simulink model "problem3model"  (R2020a)
settings: Solver=ode45  StartTime=0.0  StopTime=25  MaxStep=0.1  RelTol=1e-3  AbsTol=1e-6
PostLoadFcn:
  | g = 32.18;
  | v0 = 88;
  | Rr = 15/12;  % Wheel radius
  | Kf = 1;
  | m = 50;
  | PBmax = 1500;
  | TB = 0.01;
  | I = 5;
undefined symbols (not defined in the file): mu, sigbuilder_block, slip
settings Model: Creator=Jake  LastModifiedBy=Jake

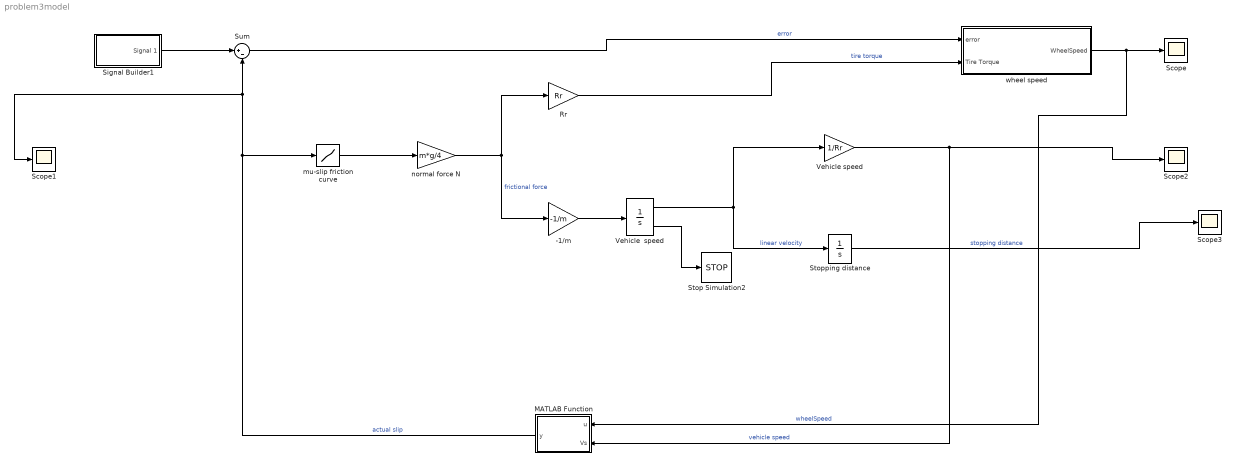
== system problem3model ==
  -1/m : Gain  Gain=-1/m  SaturateOnIntegerOverflow=on  OutDataTypeStr=Inherit: Same as input  ParamDataTypeStr=Inherit: Same as input
  MATLAB Function : MATLAB Function  TreatAsAtomicUnit=on
  Rr : Gain  Gain=Rr  SaturateOnIntegerOverflow=on  OutDataTypeStr=Inherit: Same as input  ParamDataTypeStr=Inherit: Same as input
  Scope{,1..3} (4 alike) : Scope
  Signal Builder1 : Subsystem  Tag=STV Subsys  LoadFcn=sigbuilder_block('load');  StartFcn=sigbuilder_block('start');  StopFcn=sigbuilder_block('stop');  ClipboardFcn=sigbuilder_block('clipboard');  mask(Sigbuilder block){tuvar=[0:10]}
      mask help: Simulink:masks:SigbuilderBlock_MD
      mask init:
      | if ~strcmp(get_param(bdroot(gcbh),'SimulationStatus'),'stopped') tuvar = sigbuilder_block('maskInit'); end
      settings: CopyFcn=sigbuilder_block('copy');  DeleteFcn=sigbuilder_block('delete');  ModelCloseFcn=sigbuilder_block('modelClose');  PreSaveFcn=sigbuilder_block('preSave');  PauseFcn=sigbuilder_block('pause');  ContinueFcn=sigbuilder_block('continue');  NameChangeFcn=sigbuilder_block('namechange');  OpenFcn=sigbuilder_block('open',[404 117.5 550.5 362.5 ]);  CloseFcn=sigbuilder_block('close');
      mask Display: plot(0, 0, 100, 100,[2, 2, 32, 32, 2], [68, 8, 8, 68, 68],[32, 2], [38, 38], [32, 19, 2],[53, 60, 44], [32, 17, 17, 2],[16, 16, 31, 31]);txt = getActiveGroup(gcbh);text(2, 100, txt,'verticalAlignment', 'top');
  Stop Simulation2 : Stop
  Stopping distance : Integrator  UpperSaturationLimit=1000  LowerSaturationLimit=0
  Sum : Sum  Inputs=|+-
  Vehicle  speed : Integrator  InitialCondition=v0  LimitOutput=on  UpperSaturationLimit=1000  LowerSaturationLimit=0  ShowSaturationPort=on
  Vehicle speed : Gain  Gain=1/Rr  SaturateOnIntegerOverflow=on  OutDataTypeStr=Inherit: Same as input  ParamDataTypeStr=Inherit: Same as input
  mu-slip friction curve : Lookup_n-D  NumberOfTableDimensions=1  BreakpointsForDimension1=slip  Table=mu  SaturateOnIntegerOverflow=on  InputSameDT=on
  normal force N : Gain  Gain=m*g/4
  wheel speed : Subsystem
  wires:
  Signal Builder1/1(Signal 1) -> Sum/1
  MATLAB Function/1(y) -> mu-slip friction curve/1, Scope1/1, Sum/2  "actual slip"
  normal force N/1 -> -1/m/1, Rr/1  "frictional force"
  -1/m/1 -> Vehicle  speed/1
  Vehicle  speed/2 -> Stop Simulation2/1
  Vehicle  speed/1 -> Stopping distance/1, Vehicle speed/1  "linear velocity"
  Stopping distance/1 -> Scope3/1  "stopping distance"
  mu-slip friction curve/1 -> normal force N/1
  Vehicle speed/1 -> MATLAB Function/2(Vs), Scope2/1  "vehicle speed"
  Sum/1 -> wheel speed/1(error)  "error"
  Rr/1 -> wheel speed/2(Tire Torque)  "tire torque"
  wheel speed/1(WheelSpeed) -> MATLAB Function/1(u), Scope/1  "wheelSpeed"

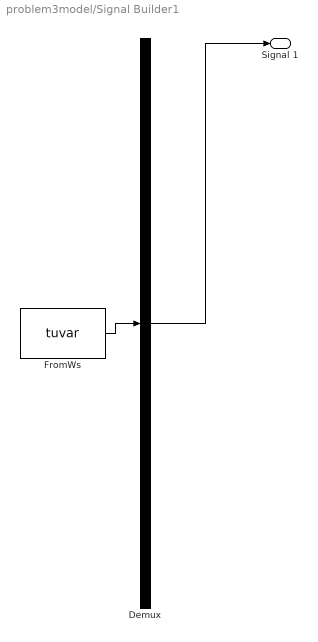
== system problem3model/Signal Builder1 ==
  Demux : Demux  Tag=STV Demux  Outputs=1
      settings: DisplayOption=none
  FromWs : FromWorkspace  Tag=STV FromWs  VariableName=tuvar
      SigBuilderData=|
      | common.afterFinalStr = 'Extrapolate'
      | common.sampleTime = 0
      | dataSet.timeRange = [0 50]
      | dataSet.name = 'Group 1'
      | sbobj.Groups.Name = 'Group 1'
      | sbobj.Groups.Signals.Name = 'Signal 1'
      | sbobj.Groups.Signals.XData = [0 4 6 50]
      | sbobj.Groups.Signals.YData = [0.2 0.2 0.2 0.2]
      | sbobj.Groups.TimeRange = [0 50]
  Signal 1 : Outport  Tag=STV Outport
  wires:
  Demux/1 -> Signal 1/1
  FromWs/1 -> Demux/1

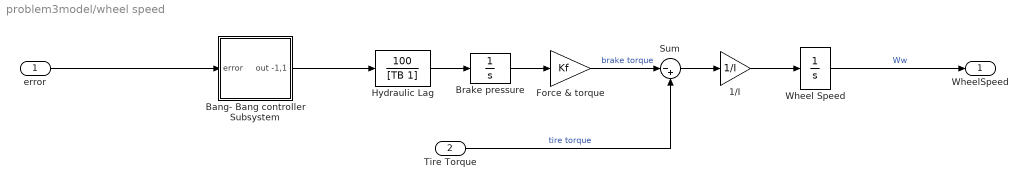
== system problem3model/wheel speed ==
  error : Inport
  Tire Torque : Inport  Port=2
  "  Bang- Bang controller Subsystem" : Subsystem
  1/I : Gain  Gain=1/I  SaturateOnIntegerOverflow=on  OutDataTypeStr=Inherit: Same as input  ParamDataTypeStr=Inherit: Same as input
  Brake pressure : Integrator  LimitOutput=on  UpperSaturationLimit=PBmax  LowerSaturationLimit=0
  Force & torque : Gain  Gain=Kf  SaturateOnIntegerOverflow=on  OutDataTypeStr=Inherit: Same as input  ParamDataTypeStr=Inherit: Same as input
  "Hydraulic Lag " : TransferFcn  Numerator=[100]  Denominator=[TB 1]
  Sum : Sum  Inputs=|-+  InputSameDT=on  SaturateOnIntegerOverflow=on  OutDataTypeStr=Inherit: Same as first input
  Wheel Speed : Integrator  InitialCondition=v0/Rr  LimitOutput=on  UpperSaturationLimit=1000  LowerSaturationLimit=0
  WheelSpeed : Outport  VectorParamsAs1DForOutWhenUnconnected=off
  wires:
  error/1 -> "  Bang- Bang controller Subsystem"/1(error)
  Wheel Speed/1 -> WheelSpeed/1  "Ww"
  Sum/1 -> 1/I/1
  Brake pressure/1 -> Force & torque/1
  Force & torque/1 -> Sum/1  "brake torque"
  "Hydraulic Lag "/1 -> Brake pressure/1
  "  Bang- Bang controller Subsystem"/1(out -1,1) -> "Hydraulic Lag "/1
  Tire Torque/1 -> Sum/2  "tire torque"
  1/I/1 -> Wheel Speed/1

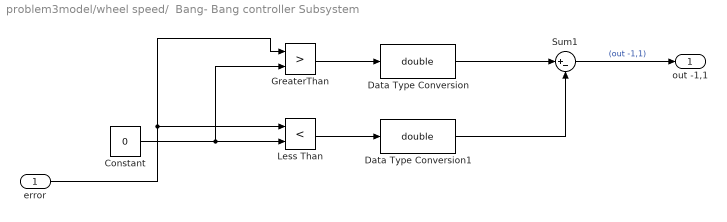
== system problem3model/wheel speed/  Bang- Bang controller Subsystem ==
  error : Inport  SampleTime=0
  Constant : Constant  Value=0
  Data Type Conversion : DataTypeConversion  OutDataTypeStr=double  RndMeth=Zero
  Data Type Conversion1 : DataTypeConversion  OutDataTypeStr=double  RndMeth=Zero
  GreaterThan : RelationalOperator  Operator=>  OutDataTypeStr=boolean  RndMeth=Simplest
  Less Than : RelationalOperator  Operator=<  OutDataTypeStr=boolean  RndMeth=Simplest
  Sum1 : Sum  Inputs=|+-
  out -1,1 : Outport
  wires:
  Sum1/1 -> out -1,1/1  "(out -1,1)"
  Less Than/1 -> Data Type Conversion1/1
  GreaterThan/1 -> Data Type Conversion/1
  Data Type Conversion/1 -> Sum1/1
  error/1 -> GreaterThan/1, Less Than/1
  Constant/1 -> GreaterThan/2, Less Than/2
  Data Type Conversion1/1 -> Sum1/2

== matlab function problem3model/MATLAB Function ==
  data: u input; y output; Vs input
function y = fcn(u,Vs)

y = 1.0-u/(Vs+(Vs==0)*eps);
